simulink model "E010A5_R2_E3_scheduler_release_40A_1A_20260701_003900"  (R2024b)
settings: Solver=VariableStepAuto  StartTime=0.0  StopTime=0.54e-3  MaxStep=5e-9  RelTol=1e-3
undefined symbols (not defined in the file): A_init, A_lower, A_upper, Cout, DCR_L1, DCR_L2, DCR_L3, DCR_L4, E010_AreaBleed_Enable, E010_AreaHold_Enable, E010_AreaHold_Time, E010_PulseInhibit_Count, E010_PulseInhibit_Enable, E010_PulseInhibit_Time, E010_Reentry_Band_Down, E010_ReentryGuard_Enable, E010_TonTrunc_Enable, E010_Vref, E010A5_DeltaI_Drop_Threshold_High, E010A5_IL_Sense_Gain1, E010A5_IL_Sense_Gain2, E010A5_IL_Sense_Gain3, E010A5_IL_Sense_Gain4, E010A5_R2_BudgetWindow, E010A5_R2_EnergyShaper_Enable, E010A5_R2_FirstTonLimit, E010A5_R2_PreloadTarget, E010A5_R2_ReleaseInitial, E010A5_R2_ReleaseRate, E010A5_R2_ReleaseWindow, E010A5_R2_RestoreRate, E010A5_R2_SchedulerGateEnable, E010A5_R2_SchedulerReleaseEnable, E010A5_R2_SecondTonLimit, E010A5_R2_SoftPreloadEnable, E010A5_R2_TonBudget, E010A5_R2_TonRampMax, E010A5_R2_TonRampStep, E010A5_R2_TonRampWindow, E010A5_R2_UndershootBudget, E010A5_R2_UpperReentryBand, E010A5_R2_VoltageWindowEnable, ESR_C, IdealIQCOT_Enable, IL_adc_counts_per_A, IL_pk_limit_adc_neg, IL_pk_limit_adc_pos, Iload_final, Iload_initial, Iph, Iqcot_enable, kappa_cmd, Kiqcot, Kvc_iqcot, L, Lambda0_iqcot, Lambda_m2, rho_cmd, Ri_iqcot, t_load_step ... (+19)
libraries: simulink x29, spsCurrentMeasurementLib x8, spsMosfetLib x8, spsSeriesRLCBranchLib x5, spsVoltageMeasurementLib x5, spsDCVoltageSourceLib x4, spsControlledCurrentSourceLib x1, spsGroundLib x1, spspowerguiLib x1
(part 2 of 2)

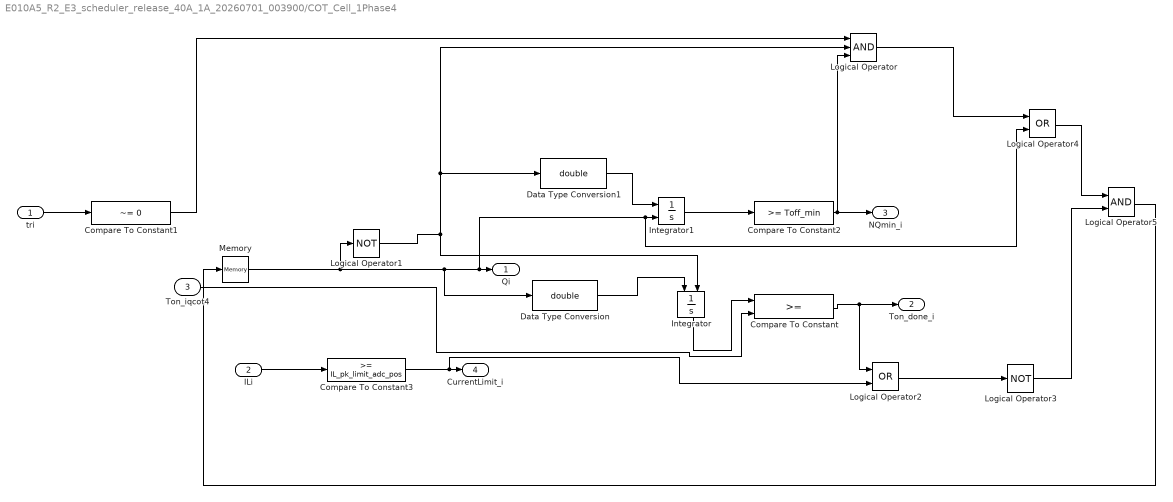
== system E010A5_R2_E3_scheduler_release_40A_1A_20260701_003900/COT_Cell_1Phase4 ==
  tri : Inport
  ILi : Inport  Port=2
  Ton_iqcot4 : Inport  Port=3
  Compare To Constant : RelationalOperator  OutDataTypeStr=boolean  RndMeth=Simplest  InputSameDT=off
  Compare To Constant1 : simulink/Logic and Bit Operations/Compare To Constant  relop=~=  const=0  OutDataTypeStr=boolean
  Compare To Constant2 : simulink/Logic and Bit Operations/Compare To Constant  relop=>=  const=Toff_min  OutDataTypeStr=boolean
  Compare To Constant3 : simulink/Logic and Bit Operations/Compare To Constant  relop=>=  const=IL_pk_limit_adc_pos  OutDataTypeStr=boolean
  Data Type Conversion : DataTypeConversion  OutDataTypeStr=double  SaturateOnIntegerOverflow=off  RndMeth=Floor
  Data Type Conversion1 : DataTypeConversion  OutDataTypeStr=double  SaturateOnIntegerOverflow=off  RndMeth=Floor
  Integrator : Integrator  ExternalReset=level
  Integrator1 : Integrator  ExternalReset=level  InitialCondition=Toff_min
  Logical Operator : Logic  Inputs=3  AllPortsSameDT=off  OutDataTypeStr=boolean
  Logical Operator1 : Logic  Operator=NOT  AllPortsSameDT=off  OutDataTypeStr=boolean
  Logical Operator2 : Logic  Operator=OR  AllPortsSameDT=off  OutDataTypeStr=boolean
  Logical Operator3 : Logic  Operator=NOT  Inputs=3  AllPortsSameDT=off  OutDataTypeStr=boolean
  Logical Operator4 : Logic  Operator=OR  AllPortsSameDT=off  OutDataTypeStr=boolean
  Logical Operator5 : Logic  AllPortsSameDT=off  OutDataTypeStr=boolean
  Memory : Memory
  Qi : Outport
  Ton_done_i : Outport  Port=2
  NQmin_i : Outport  Port=3
  CurrentLimit_i : Outport  Port=4
  wires:
  Compare To Constant/1 -> Logical Operator2/1, Ton_done_i/1
  tri/1 -> Compare To Constant1/1
  Compare To Constant1/1 -> Logical Operator/1
  Memory/1 -> Logical Operator1/1, Data Type Conversion/1, Logical Operator4/2, Integrator1/2, Qi/1
  Logical Operator1/1 -> Data Type Conversion1/1, Logical Operator/2, Integrator/2
  Data Type Conversion/1 -> Integrator/1
  Integrator/1 -> Compare To Constant/1
  Data Type Conversion1/1 -> Integrator1/1
  Integrator1/1 -> Compare To Constant2/1
  Compare To Constant2/1 -> Logical Operator/3, NQmin_i/1
  ILi/1 -> Compare To Constant3/1
  Compare To Constant3/1 -> Logical Operator2/2, CurrentLimit_i/1
  Logical Operator2/1 -> Logical Operator3/1
  Logical Operator/1 -> Logical Operator4/1
  Logical Operator4/1 -> Logical Operator5/1
  Logical Operator3/1 -> Logical Operator5/2
  Logical Operator5/1 -> Memory/1
  Ton_iqcot4/1 -> Compare To Constant/2

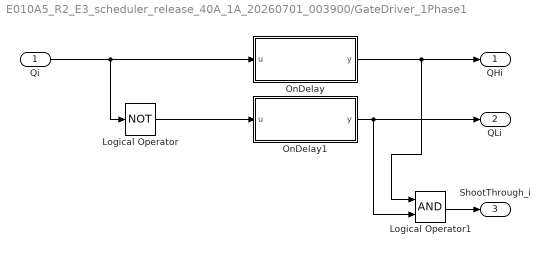
== system E010A5_R2_E3_scheduler_release_40A_1A_20260701_003900/GateDriver_1Phase1 ==
  Qi : Inport
  Logical Operator : Logic  Operator=NOT  AllPortsSameDT=off  OutDataTypeStr=boolean
  Logical Operator1 : Logic  AllPortsSameDT=off  OutDataTypeStr=boolean
  OnDelay : Subsystem
  OnDelay1 : Subsystem
  QHi : Outport
  QLi : Outport  Port=2
  ShootThrough_i : Outport  Port=3
  wires:
  Qi/1 -> Logical Operator/1, OnDelay/1(u)
  OnDelay/1(y) -> Logical Operator1/1, QHi/1
  Logical Operator/1 -> OnDelay1/1(u)
  OnDelay1/1(y) -> QLi/1, Logical Operator1/2
  Logical Operator1/1 -> ShootThrough_i/1

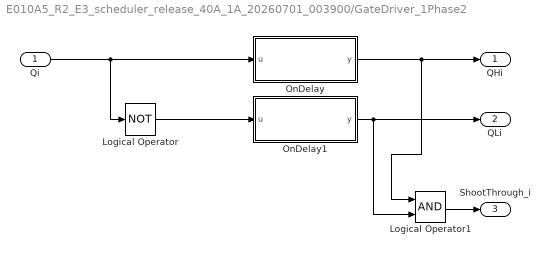
== system E010A5_R2_E3_scheduler_release_40A_1A_20260701_003900/GateDriver_1Phase2 ==
  Qi : Inport
  Logical Operator : Logic  Operator=NOT  AllPortsSameDT=off  OutDataTypeStr=boolean
  Logical Operator1 : Logic  AllPortsSameDT=off  OutDataTypeStr=boolean
  OnDelay : Subsystem
  OnDelay1 : Subsystem
  QHi : Outport
  QLi : Outport  Port=2
  ShootThrough_i : Outport  Port=3
  wires:
  Qi/1 -> Logical Operator/1, OnDelay/1(u)
  OnDelay/1(y) -> Logical Operator1/1, QHi/1
  Logical Operator/1 -> OnDelay1/1(u)
  OnDelay1/1(y) -> QLi/1, Logical Operator1/2
  Logical Operator1/1 -> ShootThrough_i/1

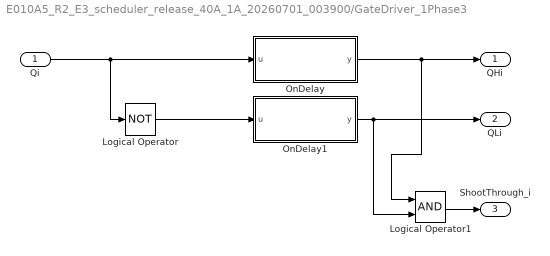
== system E010A5_R2_E3_scheduler_release_40A_1A_20260701_003900/GateDriver_1Phase3 ==
  Qi : Inport
  Logical Operator : Logic  Operator=NOT  AllPortsSameDT=off  OutDataTypeStr=boolean
  Logical Operator1 : Logic  AllPortsSameDT=off  OutDataTypeStr=boolean
  OnDelay : Subsystem
  OnDelay1 : Subsystem
  QHi : Outport
  QLi : Outport  Port=2
  ShootThrough_i : Outport  Port=3
  wires:
  Qi/1 -> Logical Operator/1, OnDelay/1(u)
  OnDelay/1(y) -> Logical Operator1/1, QHi/1
  Logical Operator/1 -> OnDelay1/1(u)
  OnDelay1/1(y) -> QLi/1, Logical Operator1/2
  Logical Operator1/1 -> ShootThrough_i/1

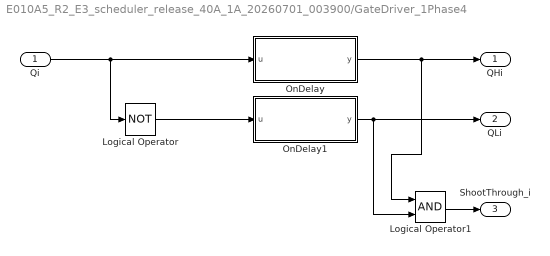
== system E010A5_R2_E3_scheduler_release_40A_1A_20260701_003900/GateDriver_1Phase4 ==
  Qi : Inport
  Logical Operator : Logic  Operator=NOT  AllPortsSameDT=off  OutDataTypeStr=boolean
  Logical Operator1 : Logic  AllPortsSameDT=off  OutDataTypeStr=boolean
  OnDelay : Subsystem
  OnDelay1 : Subsystem
  QHi : Outport
  QLi : Outport  Port=2
  ShootThrough_i : Outport  Port=3
  wires:
  Qi/1 -> Logical Operator/1, OnDelay/1(u)
  OnDelay/1(y) -> Logical Operator1/1, QHi/1
  Logical Operator/1 -> OnDelay1/1(u)
  OnDelay1/1(y) -> QLi/1, Logical Operator1/2
  Logical Operator1/1 -> ShootThrough_i/1

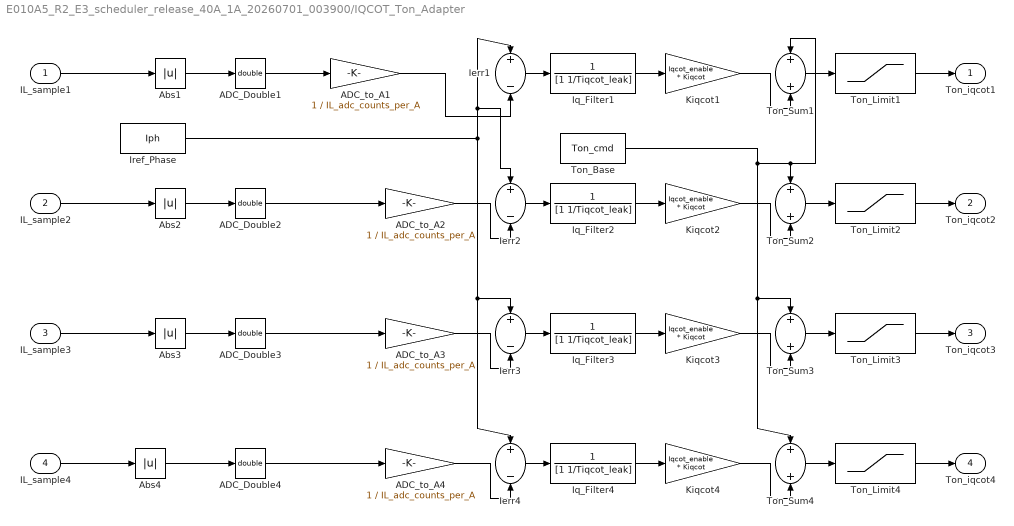
== system E010A5_R2_E3_scheduler_release_40A_1A_20260701_003900/IQCOT_Ton_Adapter ==
  IL_sample1 : Inport
  IL_sample2 : Inport  Port=2
  IL_sample3 : Inport  Port=3
  IL_sample4 : Inport  Port=4
  ADC_Double{1..4} (4 alike) : DataTypeConversion  OutDataTypeStr=double  SaturateOnIntegerOverflow=off  RndMeth=Floor
  ADC_to_A{1..4} (4 alike) : Gain  Gain=1 / IL_adc_counts_per_A  OutDataTypeStr=double
  Abs{1..4} (4 alike) : Abs  SaturateOnIntegerOverflow=off
  Ierr{1..4} (4 alike) : Sum  Inputs=+-
  Iq_Filter{1..4} (4 alike) : TransferFcn  Numerator=1  Denominator=[1 1/Tiqcot_leak]
  Iref_Phase : Constant  Value=Iph
  Kiqcot{1..4} (4 alike) : Gain  Gain=Iqcot_enable * Kiqcot
  Ton_Base : Constant  Value=Ton_cmd
  Ton_Limit{1..4} (4 alike) : Saturate  UpperLimit=Ton_iq_max  LowerLimit=Ton_iq_min
  Ton_Sum{1..4} (4 alike) : Sum
  Ton_iqcot1 : Outport
  Ton_iqcot2 : Outport  Port=2
  Ton_iqcot3 : Outport  Port=3
  Ton_iqcot4 : Outport  Port=4
  wires:
  IL_sample1/1 -> Abs1/1
  Abs1/1 -> ADC_Double1/1
  ADC_to_A1/1 -> Ierr1/2
  Iref_Phase/1 -> Ierr1/1, Ierr2/1, Ierr3/1, Ierr4/1
  Ierr1/1 -> Iq_Filter1/1
  Iq_Filter1/1 -> Kiqcot1/1
  Kiqcot1/1 -> Ton_Sum1/2
  Ton_Base/1 -> Ton_Sum3/1, Ton_Sum4/1, Ton_Sum1/1, Ton_Sum2/1
  Ton_Sum1/1 -> Ton_Limit1/1
  Ton_Limit1/1 -> Ton_iqcot1/1
  IL_sample2/1 -> Abs2/1
  Abs2/1 -> ADC_Double2/1
  ADC_to_A2/1 -> Ierr2/2
  Ierr2/1 -> Iq_Filter2/1
  Iq_Filter2/1 -> Kiqcot2/1
  Kiqcot2/1 -> Ton_Sum2/2
  Ton_Sum2/1 -> Ton_Limit2/1
  Ton_Limit2/1 -> Ton_iqcot2/1
  IL_sample3/1 -> Abs3/1
  Abs3/1 -> ADC_Double3/1
  ADC_to_A3/1 -> Ierr3/2
  Ierr3/1 -> Iq_Filter3/1
  Iq_Filter3/1 -> Kiqcot3/1
  Kiqcot3/1 -> Ton_Sum3/2
  Ton_Sum3/1 -> Ton_Limit3/1
  Ton_Limit3/1 -> Ton_iqcot3/1
  IL_sample4/1 -> Abs4/1
  Abs4/1 -> ADC_Double4/1
  ADC_to_A4/1 -> Ierr4/2
  Ierr4/1 -> Iq_Filter4/1
  Iq_Filter4/1 -> Kiqcot4/1
  Kiqcot4/1 -> Ton_Sum4/2
  Ton_Sum4/1 -> Ton_Limit4/1
  Ton_Limit4/1 -> Ton_iqcot4/1
  ADC_Double1/1 -> ADC_to_A1/1
  ADC_Double2/1 -> ADC_to_A2/1
  ADC_Double3/1 -> ADC_to_A3/1
  ADC_Double4/1 -> ADC_to_A4/1

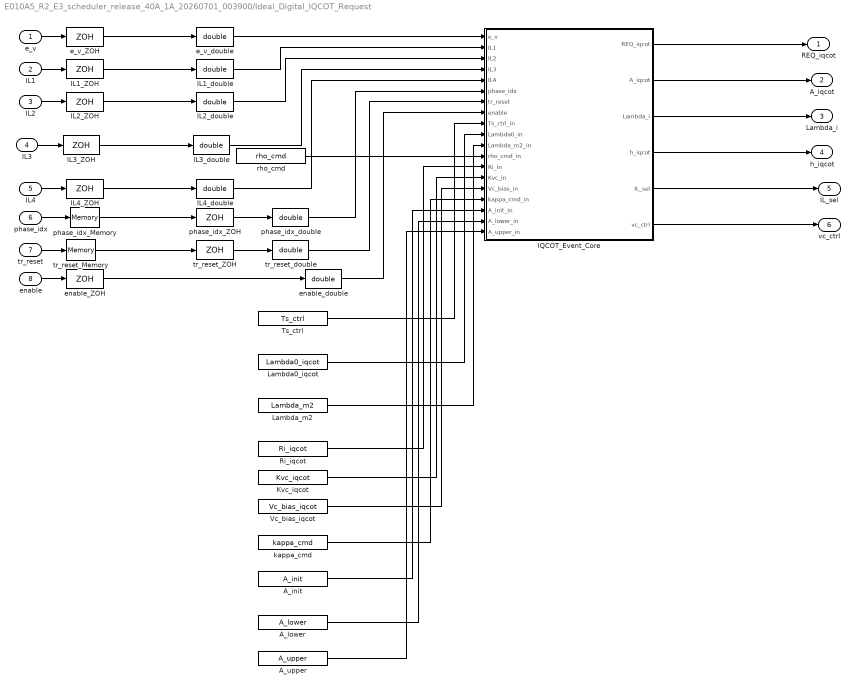
== system E010A5_R2_E3_scheduler_release_40A_1A_20260701_003900/Ideal_Digital_IQCOT_Request ==
  e_v : Inport
  IL1 : Inport  Port=2
  IL2 : Inport  Port=3
  IL3 : Inport  Port=4
  IL4 : Inport  Port=5
  phase_idx : Inport  Port=6
  tr_reset : Inport  Port=7
  enable : Inport  Port=8
  A_init : Constant  Value=A_init
  A_lower : Constant  Value=A_lower
  A_upper : Constant  Value=A_upper
  IL1_ZOH : ZeroOrderHold  SampleTime=Ts_ctrl
  IL1_double : DataTypeConversion  OutDataTypeStr=double  SaturateOnIntegerOverflow=off  RndMeth=Floor
  IL2_ZOH : ZeroOrderHold  SampleTime=Ts_ctrl
  IL2_double : DataTypeConversion  OutDataTypeStr=double  SaturateOnIntegerOverflow=off  RndMeth=Floor
  IL3_ZOH : ZeroOrderHold  SampleTime=Ts_ctrl
  IL3_double : DataTypeConversion  OutDataTypeStr=double  SaturateOnIntegerOverflow=off  RndMeth=Floor
  IL4_ZOH : ZeroOrderHold  SampleTime=Ts_ctrl
  IL4_double : DataTypeConversion  OutDataTypeStr=double  SaturateOnIntegerOverflow=off  RndMeth=Floor
  IQCOT_Event_Core : MATLAB Function  TreatAsAtomicUnit=on
  Kvc_iqcot : Constant  Value=Kvc_iqcot
  Lambda0_iqcot : Constant  Value=Lambda0_iqcot
  Lambda_m2 : Constant  Value=Lambda_m2
  Ri_iqcot : Constant  Value=Ri_iqcot
  Ts_ctrl : Constant  Value=Ts_ctrl
  Vc_bias_iqcot : Constant  Value=Vc_bias_iqcot
  e_v_ZOH : ZeroOrderHold  SampleTime=Ts_ctrl
  e_v_double : DataTypeConversion  OutDataTypeStr=double  SaturateOnIntegerOverflow=off  RndMeth=Floor
  enable_ZOH : ZeroOrderHold  SampleTime=Ts_ctrl
  enable_double : DataTypeConversion  OutDataTypeStr=double  SaturateOnIntegerOverflow=off  RndMeth=Floor
  kappa_cmd : Constant  Value=kappa_cmd
  phase_idx_Memory : Memory
  phase_idx_ZOH : ZeroOrderHold  SampleTime=Ts_ctrl
  phase_idx_double : DataTypeConversion  OutDataTypeStr=double  SaturateOnIntegerOverflow=off  RndMeth=Floor
  rho_cmd : Constant  Value=rho_cmd
  tr_reset_Memory : Memory
  tr_reset_ZOH : ZeroOrderHold  SampleTime=Ts_ctrl
  tr_reset_double : DataTypeConversion  OutDataTypeStr=double  SaturateOnIntegerOverflow=off  RndMeth=Floor
  REQ_iqcot : Outport
  A_iqcot : Outport  Port=2
  Lambda_i : Outport  Port=3
  h_iqcot : Outport  Port=4
  IL_sel : Outport  Port=5
  vc_ctrl : Outport  Port=6
  wires:
  e_v/1 -> e_v_ZOH/1
  e_v_ZOH/1 -> e_v_double/1
  IL1/1 -> IL1_ZOH/1
  IL1_ZOH/1 -> IL1_double/1
  IL2/1 -> IL2_ZOH/1
  IL2_ZOH/1 -> IL2_double/1
  IL3/1 -> IL3_ZOH/1
  IL3_ZOH/1 -> IL3_double/1
  IL4/1 -> IL4_ZOH/1
  IL4_ZOH/1 -> IL4_double/1
  phase_idx/1 -> phase_idx_Memory/1
  phase_idx_Memory/1 -> phase_idx_ZOH/1
  phase_idx_ZOH/1 -> phase_idx_double/1
  tr_reset/1 -> tr_reset_Memory/1
  tr_reset_Memory/1 -> tr_reset_ZOH/1
  tr_reset_ZOH/1 -> tr_reset_double/1
  enable/1 -> enable_ZOH/1
  enable_ZOH/1 -> enable_double/1
  e_v_double/1 -> IQCOT_Event_Core/1(e_v)
  IL1_double/1 -> IQCOT_Event_Core/2(IL1)
  IL2_double/1 -> IQCOT_Event_Core/3(IL2)
  IL3_double/1 -> IQCOT_Event_Core/4(IL3)
  IL4_double/1 -> IQCOT_Event_Core/5(IL4)
  phase_idx_double/1 -> IQCOT_Event_Core/6(phase_idx)
  tr_reset_double/1 -> IQCOT_Event_Core/7(tr_reset)
  enable_double/1 -> IQCOT_Event_Core/8(enable)
  Ts_ctrl/1 -> IQCOT_Event_Core/9(Ts_ctrl_in)
  Lambda0_iqcot/1 -> IQCOT_Event_Core/10(Lambda0_in)
  Lambda_m2/1 -> IQCOT_Event_Core/11(Lambda_m2_in)
  rho_cmd/1 -> IQCOT_Event_Core/12(rho_cmd_in)
  Ri_iqcot/1 -> IQCOT_Event_Core/13(Ri_in)
  Kvc_iqcot/1 -> IQCOT_Event_Core/14(Kvc_in)
  Vc_bias_iqcot/1 -> IQCOT_Event_Core/15(Vc_bias_in)
  kappa_cmd/1 -> IQCOT_Event_Core/16(kappa_cmd_in)
  A_init/1 -> IQCOT_Event_Core/17(A_init_in)
  A_lower/1 -> IQCOT_Event_Core/18(A_lower_in)
  A_upper/1 -> IQCOT_Event_Core/19(A_upper_in)
  IQCOT_Event_Core/1(REQ_iqcot) -> REQ_iqcot/1
  IQCOT_Event_Core/2(A_iqcot) -> A_iqcot/1
  IQCOT_Event_Core/3(Lambda_i) -> Lambda_i/1
  IQCOT_Event_Core/4(h_iqcot) -> h_iqcot/1
  IQCOT_Event_Core/5(IL_sel) -> IL_sel/1
  IQCOT_Event_Core/6(vc_ctrl) -> vc_ctrl/1

== system E010A5_R2_E3_scheduler_release_40A_1A_20260701_003900/OnDelay ==
  u : Inport
  Compare To Constant : simulink/Logic and Bit Operations/Compare To Constant  relop=>=  const=Tdead  OutDataTypeStr=boolean
  Data Type Conversion : DataTypeConversion  OutDataTypeStr=double  SaturateOnIntegerOverflow=off  RndMeth=Floor
  Integrator : Integrator  ExternalReset=level
  Logical Operator : Logic  Operator=NOT  AllPortsSameDT=off  OutDataTypeStr=boolean
  y : Outport
  wires:
  u/1 -> Data Type Conversion/1, Logical Operator/1
  Logical Operator/1 -> Integrator/2
  Data Type Conversion/1 -> Integrator/1
  Integrator/1 -> Compare To Constant/1
  Compare To Constant/1 -> y/1

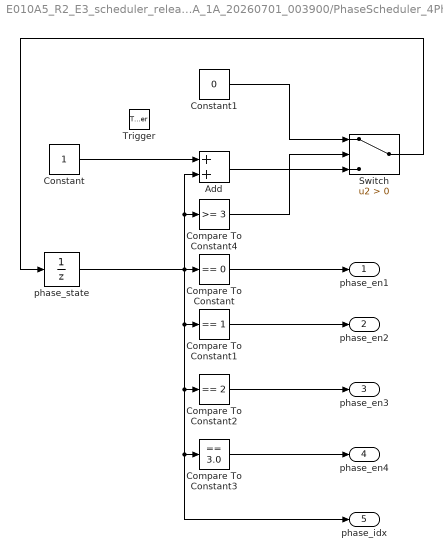
== system E010A5_R2_E3_scheduler_release_40A_1A_20260701_003900/PhaseScheduler_4Phase ==
  Trigger : TriggerPort  VariantControl=(inherit)
  Add : Sum
  Compare To Constant : simulink/Logic and Bit Operations/Compare To Constant  relop===  const=0  OutDataTypeStr=boolean
  Compare To Constant1 : simulink/Logic and Bit Operations/Compare To Constant  relop===  const=1  OutDataTypeStr=boolean
  Compare To Constant2 : simulink/Logic and Bit Operations/Compare To Constant  relop===  const=2  OutDataTypeStr=boolean
  Compare To Constant3 : simulink/Logic and Bit Operations/Compare To Constant  relop===  const=3.0  OutDataTypeStr=boolean
  Compare To Constant4 : simulink/Logic and Bit Operations/Compare To Constant  relop=>=  const=3  OutDataTypeStr=boolean
  Constant : Constant
  Constant1 : Constant  Value=0
  Switch : Switch  Criteria=u2 > Threshold  SaturateOnIntegerOverflow=off  InputSameDT=off
  phase_state : UnitDelay  SampleTime=-1  HasFrameUpgradeWarning=on
  phase_en1 : Outport
  phase_en2 : Outport  Port=2
  phase_en3 : Outport  Port=3
  phase_en4 : Outport  Port=4
  phase_idx : Outport  Port=5
  wires:
  phase_state/1 -> phase_idx/1, Compare To Constant3/1, Compare To Constant2/1, Compare To Constant1/1, Compare To Constant/1, Compare To Constant4/1, Add/2
  Compare To Constant/1 -> phase_en1/1
  Compare To Constant1/1 -> phase_en2/1
  Compare To Constant2/1 -> phase_en3/1
  Compare To Constant3/1 -> phase_en4/1
  Constant/1 -> Add/1
  Add/1 -> Switch/3
  Compare To Constant4/1 -> Switch/2
  Constant1/1 -> Switch/1
  Switch/1 -> phase_state/1

== system E010A5_R2_E3_scheduler_release_40A_1A_20260701_003900/GateDriver_1Phase1/OnDelay ==
  u : Inport
  Compare To Constant : simulink/Logic and Bit Operations/Compare To Constant  relop=>=  const=Tdead  OutDataTypeStr=boolean
  Data Type Conversion : DataTypeConversion  OutDataTypeStr=double  SaturateOnIntegerOverflow=off  RndMeth=Floor
  Integrator : Integrator  ExternalReset=level
  Logical Operator : Logic  Operator=NOT  AllPortsSameDT=off  OutDataTypeStr=boolean
  y : Outport
  wires:
  u/1 -> Data Type Conversion/1, Logical Operator/1
  Logical Operator/1 -> Integrator/2
  Data Type Conversion/1 -> Integrator/1
  Integrator/1 -> Compare To Constant/1
  Compare To Constant/1 -> y/1

== system E010A5_R2_E3_scheduler_release_40A_1A_20260701_003900/GateDriver_1Phase1/OnDelay1 ==
  u : Inport
  Compare To Constant : simulink/Logic and Bit Operations/Compare To Constant  relop=>=  const=Tdead  OutDataTypeStr=boolean
  Data Type Conversion : DataTypeConversion  OutDataTypeStr=double  SaturateOnIntegerOverflow=off  RndMeth=Floor
  Integrator : Integrator  ExternalReset=level
  Logical Operator : Logic  Operator=NOT  AllPortsSameDT=off  OutDataTypeStr=boolean
  y : Outport
  wires:
  u/1 -> Data Type Conversion/1, Logical Operator/1
  Logical Operator/1 -> Integrator/2
  Data Type Conversion/1 -> Integrator/1
  Integrator/1 -> Compare To Constant/1
  Compare To Constant/1 -> y/1

== system E010A5_R2_E3_scheduler_release_40A_1A_20260701_003900/GateDriver_1Phase2/OnDelay ==
  u : Inport
  Compare To Constant : simulink/Logic and Bit Operations/Compare To Constant  relop=>=  const=Tdead  OutDataTypeStr=boolean
  Data Type Conversion : DataTypeConversion  OutDataTypeStr=double  SaturateOnIntegerOverflow=off  RndMeth=Floor
  Integrator : Integrator  ExternalReset=level
  Logical Operator : Logic  Operator=NOT  AllPortsSameDT=off  OutDataTypeStr=boolean
  y : Outport
  wires:
  u/1 -> Data Type Conversion/1, Logical Operator/1
  Logical Operator/1 -> Integrator/2
  Data Type Conversion/1 -> Integrator/1
  Integrator/1 -> Compare To Constant/1
  Compare To Constant/1 -> y/1

== system E010A5_R2_E3_scheduler_release_40A_1A_20260701_003900/GateDriver_1Phase2/OnDelay1 ==
  u : Inport
  Compare To Constant : simulink/Logic and Bit Operations/Compare To Constant  relop=>=  const=Tdead  OutDataTypeStr=boolean
  Data Type Conversion : DataTypeConversion  OutDataTypeStr=double  SaturateOnIntegerOverflow=off  RndMeth=Floor
  Integrator : Integrator  ExternalReset=level
  Logical Operator : Logic  Operator=NOT  AllPortsSameDT=off  OutDataTypeStr=boolean
  y : Outport
  wires:
  u/1 -> Data Type Conversion/1, Logical Operator/1
  Logical Operator/1 -> Integrator/2
  Data Type Conversion/1 -> Integrator/1
  Integrator/1 -> Compare To Constant/1
  Compare To Constant/1 -> y/1

== system E010A5_R2_E3_scheduler_release_40A_1A_20260701_003900/GateDriver_1Phase3/OnDelay ==
  u : Inport
  Compare To Constant : simulink/Logic and Bit Operations/Compare To Constant  relop=>=  const=Tdead  OutDataTypeStr=boolean
  Data Type Conversion : DataTypeConversion  OutDataTypeStr=double  SaturateOnIntegerOverflow=off  RndMeth=Floor
  Integrator : Integrator  ExternalReset=level
  Logical Operator : Logic  Operator=NOT  AllPortsSameDT=off  OutDataTypeStr=boolean
  y : Outport
  wires:
  u/1 -> Data Type Conversion/1, Logical Operator/1
  Logical Operator/1 -> Integrator/2
  Data Type Conversion/1 -> Integrator/1
  Integrator/1 -> Compare To Constant/1
  Compare To Constant/1 -> y/1

== system E010A5_R2_E3_scheduler_release_40A_1A_20260701_003900/GateDriver_1Phase3/OnDelay1 ==
  u : Inport
  Compare To Constant : simulink/Logic and Bit Operations/Compare To Constant  relop=>=  const=Tdead  OutDataTypeStr=boolean
  Data Type Conversion : DataTypeConversion  OutDataTypeStr=double  SaturateOnIntegerOverflow=off  RndMeth=Floor
  Integrator : Integrator  ExternalReset=level
  Logical Operator : Logic  Operator=NOT  AllPortsSameDT=off  OutDataTypeStr=boolean
  y : Outport
  wires:
  u/1 -> Data Type Conversion/1, Logical Operator/1
  Logical Operator/1 -> Integrator/2
  Data Type Conversion/1 -> Integrator/1
  Integrator/1 -> Compare To Constant/1
  Compare To Constant/1 -> y/1

== system E010A5_R2_E3_scheduler_release_40A_1A_20260701_003900/GateDriver_1Phase4/OnDelay ==
  u : Inport
  Compare To Constant : simulink/Logic and Bit Operations/Compare To Constant  relop=>=  const=Tdead  OutDataTypeStr=boolean
  Data Type Conversion : DataTypeConversion  OutDataTypeStr=double  SaturateOnIntegerOverflow=off  RndMeth=Floor
  Integrator : Integrator  ExternalReset=level
  Logical Operator : Logic  Operator=NOT  AllPortsSameDT=off  OutDataTypeStr=boolean
  y : Outport
  wires:
  u/1 -> Data Type Conversion/1, Logical Operator/1
  Logical Operator/1 -> Integrator/2
  Data Type Conversion/1 -> Integrator/1
  Integrator/1 -> Compare To Constant/1
  Compare To Constant/1 -> y/1

== system E010A5_R2_E3_scheduler_release_40A_1A_20260701_003900/GateDriver_1Phase4/OnDelay1 ==
  u : Inport
  Compare To Constant : simulink/Logic and Bit Operations/Compare To Constant  relop=>=  const=Tdead  OutDataTypeStr=boolean
  Data Type Conversion : DataTypeConversion  OutDataTypeStr=double  SaturateOnIntegerOverflow=off  RndMeth=Floor
  Integrator : Integrator  ExternalReset=level
  Logical Operator : Logic  Operator=NOT  AllPortsSameDT=off  OutDataTypeStr=boolean
  y : Outport
  wires:
  u/1 -> Data Type Conversion/1, Logical Operator/1
  Logical Operator/1 -> Integrator/2
  Data Type Conversion/1 -> Integrator/1
  Integrator/1 -> Compare To Constant/1
  Compare To Constant/1 -> y/1

== matlab function E010A5_R2_E3_scheduler_release_40A_1A_20260701_003900/E010A5_CurrentLimitHit ==
  data: u1 input boolean size=1; y output double size=1; u2 input boolean size=1; u3 input boolean size=1; u4 input boolean size=1
function y = any_four(u1,u2,u3,u4)
%#codegen
y = double((u1 > 0.5) || (u2 > 0.5) || (u3 > 0.5) || (u4 > 0.5));

== matlab function E010A5_R2_E3_scheduler_release_40A_1A_20260701_003900/E010A5_TonTrunc1 ==
  data: ton_in input double size=1; ton_out output double size=1; t input double size=1; t_step input double size=1; t_window input double size=1; t_min input double size=1; enable input double size=1; trunc_active output double size=1; ton_saved output double size=1
function [ton_out,trunc_active,ton_saved] = ton_trunc(ton_in,t,t_step,t_window,t_min,enable)
%#codegen
active = (enable > 0.5) && (t >= t_step) && (t <= (t_step + t_window));
if active
    ton_out = min(ton_in, t_min);
else
    ton_out = ton_in;
end
trunc_active = double(active);
ton_saved = max(ton_in - ton_out, 0.0);

== matlab function E010A5_R2_E3_scheduler_release_40A_1A_20260701_003900/E010A5_TonTrunc2 ==
  data: ton_in input double size=1; ton_out output double size=1; t input double size=1; t_step input double size=1; t_window input double size=1; t_min input double size=1; enable input double size=1; trunc_active output double size=1; ton_saved output double size=1
function [ton_out,trunc_active,ton_saved] = ton_trunc(ton_in,t,t_step,t_window,t_min,enable)
%#codegen
active = (enable > 0.5) && (t >= t_step) && (t <= (t_step + t_window));
if active
    ton_out = min(ton_in, t_min);
else
    ton_out = ton_in;
end
trunc_active = double(active);
ton_saved = max(ton_in - ton_out, 0.0);

== matlab function E010A5_R2_E3_scheduler_release_40A_1A_20260701_003900/E010A5_TonTrunc3 ==
  data: ton_in input double size=1; ton_out output double size=1; t input double size=1; t_step input double size=1; t_window input double size=1; t_min input double size=1; enable input double size=1; trunc_active output double size=1; ton_saved output double size=1
function [ton_out,trunc_active,ton_saved] = ton_trunc(ton_in,t,t_step,t_window,t_min,enable)
%#codegen
active = (enable > 0.5) && (t >= t_step) && (t <= (t_step + t_window));
if active
    ton_out = min(ton_in, t_min);
else
    ton_out = ton_in;
end
trunc_active = double(active);
ton_saved = max(ton_in - ton_out, 0.0);

== matlab function E010A5_R2_E3_scheduler_release_40A_1A_20260701_003900/E010A5_TonTrunc4 ==
  data: ton_in input double size=1; ton_out output double size=1; t input double size=1; t_step input double size=1; t_window input double size=1; t_min input double size=1; enable input double size=1; trunc_active output double size=1; ton_saved output double size=1
function [ton_out,trunc_active,ton_saved] = ton_trunc(ton_in,t,t_step,t_window,t_min,enable)
%#codegen
active = (enable > 0.5) && (t >= t_step) && (t <= (t_step + t_window));
if active
    ton_out = min(ton_in, t_min);
else
    ton_out = ton_in;
end
trunc_active = double(active);
ton_saved = max(ton_in - ton_out, 0.0);

== matlab function E010A5_R2_E3_scheduler_release_40A_1A_20260701_003900/E010A5_PulseInhibitState ==
  data: u1 input boolean size=1; y output double size=1; u2 input boolean size=1; u3 input boolean size=1; u4 input boolean size=1
function y = any_four(u1,u2,u3,u4)
%#codegen
y = double((u1 > 0.5) || (u2 > 0.5) || (u3 > 0.5) || (u4 > 0.5));

== matlab function E010A5_R2_E3_scheduler_release_40A_1A_20260701_003900/E010A5_PulseInhibit1 ==
  data: tr_in input boolean size=1; tr_out output boolean size=1; t input double size=1; t_step input double size=1; t_window input double size=1; count_max input double size=1; enable input double size=1; vout input double size=1; vref input double size=1; reentry_band input double size=1; guard_enable input double size=1; inhibit_active output boolean size=1; inhibit_count output double size=1
function [tr_out,inhibit_active,inhibit_count] = pulse_inhibit(tr_in,t,t_step,t_window,count_max,enable,vout,vref,reentry_band,guard_enable)
%#codegen
is_high = logical(tr_in);
in_window = (enable > 0.5) && (t >= t_step) && (t <= (t_step + t_window));
guard_ok = (guard_enable <= 0.5) || (vout >= (vref + reentry_band));
inhibit_active = is_high && in_window && (count_max > 0.0) && guard_ok;
if inhibit_active
    tr_out = false;
else
    tr_out = tr_in;
end
inhibit_count = double(inhibit_active);

== matlab function E010A5_R2_E3_scheduler_release_40A_1A_20260701_003900/E010A5_PulseInhibit2 ==
  data: tr_in input boolean size=1; tr_out output boolean size=1; t input double size=1; t_step input double size=1; t_window input double size=1; count_max input double size=1; enable input double size=1; vout input double size=1; vref input double size=1; reentry_band input double size=1; guard_enable input double size=1; inhibit_active output boolean size=1; inhibit_count output double size=1
function [tr_out,inhibit_active,inhibit_count] = pulse_inhibit(tr_in,t,t_step,t_window,count_max,enable,vout,vref,reentry_band,guard_enable)
%#codegen
is_high = logical(tr_in);
in_window = (enable > 0.5) && (t >= t_step) && (t <= (t_step + t_window));
guard_ok = (guard_enable <= 0.5) || (vout >= (vref + reentry_band));
inhibit_active = is_high && in_window && (count_max > 0.0) && guard_ok;
if inhibit_active
    tr_out = false;
else
    tr_out = tr_in;
end
inhibit_count = double(inhibit_active);

== matlab function E010A5_R2_E3_scheduler_release_40A_1A_20260701_003900/E010A5_PulseInhibit3 ==
  data: tr_in input boolean size=1; tr_out output boolean size=1; t input double size=1; t_step input double size=1; t_window input double size=1; count_max input double size=1; enable input double size=1; vout input double size=1; vref input double size=1; reentry_band input double size=1; guard_enable input double size=1; inhibit_active output boolean size=1; inhibit_count output double size=1
function [tr_out,inhibit_active,inhibit_count] = pulse_inhibit(tr_in,t,t_step,t_window,count_max,enable,vout,vref,reentry_band,guard_enable)
%#codegen
is_high = logical(tr_in);
in_window = (enable > 0.5) && (t >= t_step) && (t <= (t_step + t_window));
guard_ok = (guard_enable <= 0.5) || (vout >= (vref + reentry_band));
inhibit_active = is_high && in_window && (count_max > 0.0) && guard_ok;
if inhibit_active
    tr_out = false;
else
    tr_out = tr_in;
end
inhibit_count = double(inhibit_active);

== matlab function E010A5_R2_E3_scheduler_release_40A_1A_20260701_003900/E010A5_PulseInhibit4 ==
  data: tr_in input boolean size=1; tr_out output boolean size=1; t input double size=1; t_step input double size=1; t_window input double size=1; count_max input double size=1; enable input double size=1; vout input double size=1; vref input double size=1; reentry_band input double size=1; guard_enable input double size=1; inhibit_active output boolean size=1; inhibit_count output double size=1
function [tr_out,inhibit_active,inhibit_count] = pulse_inhibit(tr_in,t,t_step,t_window,count_max,enable,vout,vref,reentry_band,guard_enable)
%#codegen
is_high = logical(tr_in);
in_window = (enable > 0.5) && (t >= t_step) && (t <= (t_step + t_window));
guard_ok = (guard_enable <= 0.5) || (vout >= (vref + reentry_band));
inhibit_active = is_high && in_window && (count_max > 0.0) && guard_ok;
if inhibit_active
    tr_out = false;
else
    tr_out = tr_in;
end
inhibit_count = double(inhibit_active);

== matlab function E010A5_R2_E3_scheduler_release_40A_1A_20260701_003900/E010A5_AreaHold_EnableProjection ==
  data: enable_in input double size=1; enable_out output double size=1; t input double size=1; t_step input double size=1; t_hold input double size=1; hold_enable input double size=1; vout input double size=1; vref input double size=1; reentry_band input double size=1; bleed_enable input double size=1; hold_state output double size=1; hold_count output double size=1; reset_count output double size=1; bleed_count output double size=1; reentry_state output double size=1
function [enable_out,hold_state,hold_count,reset_count,bleed_count,reentry_state] = area_hold_enable(enable_in,t,t_step,t_hold,hold_enable,vout,vref,reentry_band,bleed_enable)
%#codegen
persistent was_hold reset_seen
if isempty(was_hold)
    was_hold = false;
end
if isempty(reset_seen)
    reset_seen = 0.0;
end
if t < t_step
    was_hold = false;
    reset_seen = 0.0;
end
in_window = (hold_enable > 0.5) && (t >= t_step) && (t <= (t_step + t_hold));
release_not_safe = vout >= (vref + reentry_band);
hold = in_window && release_not_safe;
enable_out = double(enable_in > 0.5);
if hold
    enable_out = 0.0;
end
hold_state = double(hold);
hold_count = double(hold);
bleed_count = double(hold && (bleed_enable > 0.5));
release_edge = (~hold) && was_hold;
if release_edge
    reset_seen = reset_seen + 1.0;
end
reset_count = reset_seen;
reentry_state = double((hold_enable > 0.5) && (t > t_step) && ~hold);
was_hold = hold;

== matlab function E010A5_R2_E3_scheduler_release_40A_1A_20260701_003900/E010A5_R2_EnergyShaper ==
  data: ton1 input double size=1; ton1o output double size=1; ton2 input double size=1; ton3 input double size=1; ton4 input double size=1; t input double size=1; t_step input double size=1; enable input double size=1; budget_window input double size=1; ton_budget input double size=1; first_lim input double size=1; second_lim input double size=1; ton_step input double size=1; ramp_window input double size=1; max_ton input double size=1; soft_enable input double size=1; preload_target input double size=1; restore_rate input double size=1; sched_enable input double size=1; release_initial input double size=1; release_rate input double size=1; release_window input double size=1; voltage_enable input double size=1; vout input double size=1; vref input double size=1; upper_band input double size=1; undershoot_budget input double size=1; req1 input boolean size=1; req2 input boolean size=1; req3 input boolean size=1; req4 input boolean size=1; ton2o output double size=1; ton3o output double size=1; ton4o output double size=1; u1 output double size=1; u2 output double size=1; u3 output double size=1; u4 output double size=1; l1 output double size=1; l2 output double size=1; l3 output double size=1; l4 output double size=1; ton_state output double size=1; budget_state output double size=1; budget_used output double size=1; budget_remaining output double size=1; budget_violation output double size=1; soft_state output double size=1; soft_count output double size=1; restore_state output double size=1; sched_state output double size=1; sched_fraction output double size=1; sched_guard_violation output double size=1; voltage_state output double size=1; voltage_violation output double size=1; controlled_active output double size=1
function [ton1o,ton2o,ton3o,ton4o,u1,u2,u3,u4,l1,l2,l3,l4,ton_state,budget_state,budget_used,budget_remaining,budget_violation,soft_state,soft_count,restore_state,sched_state,sched_fraction,sched_guard_violation,voltage_state,voltage_violation,controlled_active] = r2_energy_shaper(ton1,ton2,ton3,ton4,t,t_step,enable,budget_window,ton_budget,first_lim,second_lim,ton_step,ramp_window,max_ton,soft_enable,preload_target,restore_rate,sched_enable,release_initial,release_rate,release_window,voltage_enable,vout,vref,upper_band,undershoot_budget,req1,req2,req3,req4)
%#codegen
persistent prev_req count used first_time soft_seen
if isempty(prev_req)
    prev_req = [false,false,false,false];
end
if isempty(count)
    count = 0.0;
end
if isempty(used)
    used = 0.0;
end
if isempty(first_time)
    first_time = -1.0;
end
if isempty(soft_seen)
    soft_seen = 0.0;
end
if t < t_step
    prev_req = [false,false,false,false];
    count = 0.0;
    used = 0.0;
    first_time = -1.0;
    soft_seen = 0.0;
end
tons = [ton1,ton2,ton3,ton4];
req = [req1,req2,req3,req4] > 0.5;
rise = req & ~prev_req;
active = (enable > 0.5) && (t >= t_step);
if active && (first_time < 0.0) && any(rise)
    first_time = t;
end
if first_time >= 0.0
    age = max(t - first_time, 0.0);
else
    age = 0.0;
end
in_window = active && (first_time >= 0.0) && (age <= max(budget_window, 0.0));
if voltage_enable > 0.5
    if vout < vref - max(undershoot_budget, 0.0)
        voltage_state = 2.0;
    elseif vout > vref + max(upper_band, 0.0)
        voltage_state = 3.0;
    else
        voltage_state = 1.0;
    end
else
    voltage_state = 0.0;
end
if (sched_enable > 0.5) && in_window
    sched_fraction = min(1.0, max(0.0, release_initial) + max(age, 0.0) * max(release_rate, 0.0));
    if age > max(release_window, 0.0)
        sched_fraction = 1.0;
    end
    sched_state = 1.0 + double(sched_fraction >= 0.999);
else
    sched_fraction = 1.0;
    sched_state = 0.0;
end
if ramp_window > 0.0
    alpha = min(max(age / ramp_window, 0.0), 1.0);
else
    alpha = 1.0;
end
base_limit = first_lim + alpha * max(max_ton - first_lim, 0.0);
event_limit = first_lim;
if count >= 0.5
    event_limit = second_lim;
end
if count >= 1.5
    event_limit = second_lim + (count - 1.0) * max(ton_step, 0.0);
end
limit = min(max_ton, max(first_lim, min(base_limit, event_limit)));
if sched_enable > 0.5
    limit = max(first_lim, limit * max(sched_fraction, 0.25));
end
if voltage_state == 2.0
    limit = max_ton;
elseif voltage_state == 3.0
    limit = min(limit, first_lim);
end
outs = tons;
limits = max_ton * ones(1,4);
if in_window
    limits = limit * ones(1,4);
    for idx = 1:4
        if rise(idx)
            remaining = max(ton_budget - used, 0.0);
            allowed = min(tons(idx), limit);
            if remaining > 0.0
                allowed = min(allowed, remaining);
                allowed = max(allowed, min(first_lim, remaining));
            else
                allowed = min(allowed, first_lim);
            end
            outs(idx) = allowed;
            used = used + max(allowed, 0.0);
            count = count + 1.0;
        else
            outs(idx) = min(tons(idx), limit);
        end
    end
end
budget_remaining = max(ton_budget - used, 0.0);
budget_violation = double(in_window && (used > ton_budget + 1.0e-12));
budget_used = used;
if ~active
    ton_state = 0.0;
elseif in_window
    ton_state = 1.0;
else
    ton_state = 2.0;
end
if ~active
    budget_state = 0.0;
elseif budget_violation > 0.5
    budget_state = 3.0;
elseif in_window
    budget_state = 1.0;
else
    budget_state = 2.0;
end
soft_state = double(in_window && (soft_enable > 0.5));
if soft_state > 0.5
    soft_seen = 1.0;
end
soft_count = soft_seen;
restore_state = double((soft_seen > 0.5) && (restore_rate >= 0.0));
sched_guard_violation = double((sched_enable > 0.5) && in_window && sched_fraction < 0.249);
voltage_violation = double((voltage_enable > 0.5) && (voltage_state == 3.0));
controlled_active = double(in_window);
u = max(tons - outs, 0.0);
ton1o = outs(1); ton2o = outs(2); ton3o = outs(3); ton4o = outs(4);
u1 = u(1); u2 = u(2); u3 = u(3); u4 = u(4);
l1 = limits(1); l2 = limits(2); l3 = limits(3); l4 = limits(4);
prev_req = req;
unused_preload = preload_target; %#ok<NASGU>

== matlab function E010A5_R2_E3_scheduler_release_40A_1A_20260701_003900/E010A5_R2_FinalReqGate1 ==
  data: req_in input boolean size=1; req_out output boolean size=1; sched_fraction input double size=1; voltage_state input double size=1; phase_rank input double size=1; enable input double size=1; voltage_enable input double size=1; reject_reason output double size=1; gate_active output double size=1
function [req_out,reject_reason,gate_active] = r2_final_req_gate(req_in,sched_fraction,voltage_state,phase_rank,enable,voltage_enable)
%#codegen
gate_active = double(enable > 0.5);
allow_count = ceil(4.0 * min(max(sched_fraction, 0.0), 1.0));
allow_count = max(1.0, min(4.0, allow_count));
allow = (enable <= 0.5) || (phase_rank <= allow_count);
if (voltage_enable > 0.5) && (voltage_state == 2.0)
    allow = true;
end
req_out = (req_in > 0.5) && allow;
if (req_in > 0.5) && ~allow
    reject_reason = 4.0;
else
    reject_reason = 0.0;
end

== matlab function E010A5_R2_E3_scheduler_release_40A_1A_20260701_003900/E010A5_R2_FinalReqGate2 ==
  data: req_in input boolean size=1; req_out output boolean size=1; sched_fraction input double size=1; voltage_state input double size=1; phase_rank input double size=1; enable input double size=1; voltage_enable input double size=1; reject_reason output double size=1; gate_active output double size=1
function [req_out,reject_reason,gate_active] = r2_final_req_gate(req_in,sched_fraction,voltage_state,phase_rank,enable,voltage_enable)
%#codegen
gate_active = double(enable > 0.5);
allow_count = ceil(4.0 * min(max(sched_fraction, 0.0), 1.0));
allow_count = max(1.0, min(4.0, allow_count));
allow = (enable <= 0.5) || (phase_rank <= allow_count);
if (voltage_enable > 0.5) && (voltage_state == 2.0)
    allow = true;
end
req_out = (req_in > 0.5) && allow;
if (req_in > 0.5) && ~allow
    reject_reason = 4.0;
else
    reject_reason = 0.0;
end

== matlab function E010A5_R2_E3_scheduler_release_40A_1A_20260701_003900/E010A5_R2_FinalReqGate3 ==
  data: req_in input boolean size=1; req_out output boolean size=1; sched_fraction input double size=1; voltage_state input double size=1; phase_rank input double size=1; enable input double size=1; voltage_enable input double size=1; reject_reason output double size=1; gate_active output double size=1
function [req_out,reject_reason,gate_active] = r2_final_req_gate(req_in,sched_fraction,voltage_state,phase_rank,enable,voltage_enable)
%#codegen
gate_active = double(enable > 0.5);
allow_count = ceil(4.0 * min(max(sched_fraction, 0.0), 1.0));
allow_count = max(1.0, min(4.0, allow_count));
allow = (enable <= 0.5) || (phase_rank <= allow_count);
if (voltage_enable > 0.5) && (voltage_state == 2.0)
    allow = true;
end
req_out = (req_in > 0.5) && allow;
if (req_in > 0.5) && ~allow
    reject_reason = 4.0;
else
    reject_reason = 0.0;
end

== matlab function E010A5_R2_E3_scheduler_release_40A_1A_20260701_003900/E010A5_R2_FinalReqGate4 ==
  data: req_in input boolean size=1; req_out output boolean size=1; sched_fraction input double size=1; voltage_state input double size=1; phase_rank input double size=1; enable input double size=1; voltage_enable input double size=1; reject_reason output double size=1; gate_active output double size=1
function [req_out,reject_reason,gate_active] = r2_final_req_gate(req_in,sched_fraction,voltage_state,phase_rank,enable,voltage_enable)
%#codegen
gate_active = double(enable > 0.5);
allow_count = ceil(4.0 * min(max(sched_fraction, 0.0), 1.0));
allow_count = max(1.0, min(4.0, allow_count));
allow = (enable <= 0.5) || (phase_rank <= allow_count);
if (voltage_enable > 0.5) && (voltage_state == 2.0)
    allow = true;
end
req_out = (req_in > 0.5) && allow;
if (req_in > 0.5) && ~allow
    reject_reason = 4.0;
else
    reject_reason = 0.0;
end

== matlab function E010A5_R2_E3_scheduler_release_40A_1A_20260701_003900/E010A5_REQRejectReason ==
  data: r1 input boolean size=1; reason output double size=1; r2 input boolean size=1; r3 input boolean size=1; r4 input boolean size=1; a1 input boolean size=1; a2 input boolean size=1; a3 input boolean size=1; a4 input boolean size=1
function reason = req_reject_reason(r1,r2,r3,r4,a1,a2,a3,a4)
%#codegen
raw = (r1 > 0.5) || (r2 > 0.5) || (r3 > 0.5) || (r4 > 0.5);
acc = (a1 > 0.5) || (a2 > 0.5) || (a3 > 0.5) || (a4 > 0.5);
if raw && ~acc
    reason = 1.0;
else
    reason = 0.0;
end

== matlab function E010A5_R2_E3_scheduler_release_40A_1A_20260701_003900/E010A5_PhaseOrderError ==
  data: a1 input boolean size=1; err output double size=1; a2 input boolean size=1; a3 input boolean size=1; a4 input boolean size=1; t input double size=1; t_step input double size=1
function err = phase_order_error(a1,a2,a3,a4,t,t_step)
%#codegen
persistent prev expected
if isempty(prev)
    prev = [false,false,false,false];
end
if isempty(expected)
    expected = 0.0;
end
acc = [a1,a2,a3,a4] > 0.5;
rise = acc & ~prev;
err = 0.0;
if t < t_step
    expected = 0.0;
else
    for idx = 1:4
        if rise(idx)
            if expected > 0.5 && double(idx) ~= expected
                err = 1.0;
            end
            expected = double(idx + 1);
            if expected > 4.0
                expected = 1.0;
            end
        end
    end
end
prev = acc;

== matlab function E010A5_R2_E3_scheduler_release_40A_1A_20260701_003900/E010A5_SevereDropDetector ==
  data: iload input double size=1; detected output double size=1; t input double size=1; threshold input double size=1
function detected = severe_drop_detector(iload,t,threshold)
%#codegen
persistent initial_load latched
if isempty(initial_load)
    initial_load = iload;
end
if isempty(latched)
    latched = false;
end
if t < 1.0e-9
    initial_load = iload;
    latched = false;
end
if (initial_load - iload) >= threshold
    latched = true;
end
detected = double(latched);

== matlab function E010A5_R2_E3_scheduler_release_40A_1A_20260701_003900/E010A5_TonActual1 ==
  data: qh input boolean size=1; Ton_actual output double size=1; t input double size=1
function Ton_actual = ton_actual_estimator(qh, t)
%#codegen
persistent q_prev t_rise last_width
if isempty(q_prev)
    q_prev = 0.0;
end
if isempty(t_rise)
    t_rise = 0.0;
end
if isempty(last_width)
    last_width = 0.0;
end
is_high = double(qh > 0.5);
if is_high > 0.5 && q_prev <= 0.5
    t_rise = t;
elseif is_high <= 0.5 && q_prev > 0.5
    last_width = max(0.0, t - t_rise);
end
Ton_actual = last_width;
q_prev = is_high;

== matlab function E010A5_R2_E3_scheduler_release_40A_1A_20260701_003900/E010A5_TonActual2 ==
  data: qh input boolean size=1; Ton_actual output double size=1; t input double size=1
function Ton_actual = ton_actual_estimator(qh, t)
%#codegen
persistent q_prev t_rise last_width
if isempty(q_prev)
    q_prev = 0.0;
end
if isempty(t_rise)
    t_rise = 0.0;
end
if isempty(last_width)
    last_width = 0.0;
end
is_high = double(qh > 0.5);
if is_high > 0.5 && q_prev <= 0.5
    t_rise = t;
elseif is_high <= 0.5 && q_prev > 0.5
    last_width = max(0.0, t - t_rise);
end
Ton_actual = last_width;
q_prev = is_high;

== matlab function E010A5_R2_E3_scheduler_release_40A_1A_20260701_003900/E010A5_TonActual3 ==
  data: qh input boolean size=1; Ton_actual output double size=1; t input double size=1
function Ton_actual = ton_actual_estimator(qh, t)
%#codegen
persistent q_prev t_rise last_width
if isempty(q_prev)
    q_prev = 0.0;
end
if isempty(t_rise)
    t_rise = 0.0;
end
if isempty(last_width)
    last_width = 0.0;
end
is_high = double(qh > 0.5);
if is_high > 0.5 && q_prev <= 0.5
    t_rise = t;
elseif is_high <= 0.5 && q_prev > 0.5
    last_width = max(0.0, t - t_rise);
end
Ton_actual = last_width;
q_prev = is_high;

== matlab function E010A5_R2_E3_scheduler_release_40A_1A_20260701_003900/E010A5_TonActual4 ==
  data: qh input boolean size=1; Ton_actual output double size=1; t input double size=1
function Ton_actual = ton_actual_estimator(qh, t)
%#codegen
persistent q_prev t_rise last_width
if isempty(q_prev)
    q_prev = 0.0;
end
if isempty(t_rise)
    t_rise = 0.0;
end
if isempty(last_width)
    last_width = 0.0;
end
is_high = double(qh > 0.5);
if is_high > 0.5 && q_prev <= 0.5
    t_rise = t;
elseif is_high <= 0.5 && q_prev > 0.5
    last_width = max(0.0, t - t_rise);
end
Ton_actual = last_width;
q_prev = is_high;

== matlab function E010A5_R2_E3_scheduler_release_40A_1A_20260701_003900/E010A5_ActiveHSPhase ==
  data: qh1 input boolean size=1; active_phase output double size=1; qh2 input boolean size=1; qh3 input boolean size=1; qh4 input boolean size=1
function active_phase = active_hs_phase(qh1,qh2,qh3,qh4)
%#codegen
qh = [qh1, qh2, qh3, qh4] > 0.5;
active_phase = 0.0;
for idx = 1:4
    if qh(idx)
        active_phase = double(idx);
        return;
    end
end

== matlab function E010A5_R2_E3_scheduler_release_40A_1A_20260701_003900/Ideal_Digital_IQCOT_Request/IQCOT_Event_Core ==
  data: e_v input double size=1; REQ_iqcot output double size=1; IL1 input double size=1; IL2 input double size=1; IL3 input double size=1; IL4 input double size=1; phase_idx input double size=1; tr_reset input double size=1; enable input double size=1; Ts_ctrl_in input double size=1; Lambda0_in input double size=1; Lambda_m2_in input double size=1; rho_cmd_in input double size=1; Ri_in input double size=1; Kvc_in input double size=1; Vc_bias_in input double size=1; kappa_cmd_in input double size=1; A_init_in input double size=1; A_lower_in input double size=1; A_upper_in input double size=1; A_iqcot output double size=1; Lambda_i output double size=1; h_iqcot output double size=1; IL_sel output double size=1; vc_ctrl output double size=1
function [REQ_iqcot,A_iqcot,Lambda_i,h_iqcot,IL_sel,vc_ctrl] = IQCOT_Event_Core(e_v,IL1,IL2,IL3,IL4,phase_idx,tr_reset,enable,Ts_ctrl_in,Lambda0_in,Lambda_m2_in,rho_cmd_in,Ri_in,Kvc_in,Vc_bias_in,kappa_cmd_in,A_init_in,A_lower_in,A_upper_in)
%#codegen
REQ_iqcot = 0.0;
A_iqcot = 0.0;
Lambda_i = 0.0;
h_iqcot = 0.0;
IL_sel = 0.0;
vc_ctrl = 0.0;
persistent Astate reset_prev phase_prev
if isempty(Astate)
    Astate = double(A_init_in);
end
if isempty(reset_prev)
    reset_prev = 0.0;
end
if isempty(phase_prev)
    phase_prev = 0.0;
end
p = floor(double(phase_idx));
p = mod(p, 4);
if p == 0
    IL_sel = IL1;
elseif p == 1
    IL_sel = IL2;
elseif p == 2
    IL_sel = IL3;
else
    IL_sel = IL4;
end
Ri_eff = Ri_in * exp(kappa_cmd_in);
vc_ctrl = Vc_bias_in + Kvc_in * e_v;
h_iqcot = vc_ctrl - Ri_eff * IL_sel;
Lambda_i = Lambda0_in * (1 + rho_cmd_in) + Lambda_m2_in * cos(pi * p);
if Lambda_i < eps
    Lambda_i = eps;
end
A_update = Astate + Ts_ctrl_in * h_iqcot;
if A_update < A_lower_in
    A_update = A_lower_in;
end
if A_update > A_upper_in
    A_update = A_upper_in;
end
REQ_iqcot = double((enable > 0.5) && (A_update >= Lambda_i));
A_iqcot = A_update;
reset_rise = (tr_reset > 0.5) && (reset_prev <= 0.5);
phase_change = (p ~= phase_prev);
if enable <= 0.5
    Astate = A_init_in;
elseif reset_rise || phase_change
    Astate = A_init_in;
else
    Astate = A_update;
end
reset_prev = double(tr_reset);
phase_prev = p;
